simulink model "accTests"  (R2019a)
settings: Solver=VariableStepAuto  StartTime=0.0  StopTime=25  RelTol=1e-3
libraries: simulink x21, autolibshared x5
(part 1 of 2)
settings Model: Creator=Fernando VM  LastModifiedBy=fvall
settings DataIOCC: ReturnWorkspaceOutputs=off
settings DebuggingCC: ArithmeticOperatorsInVariantConditions=warning

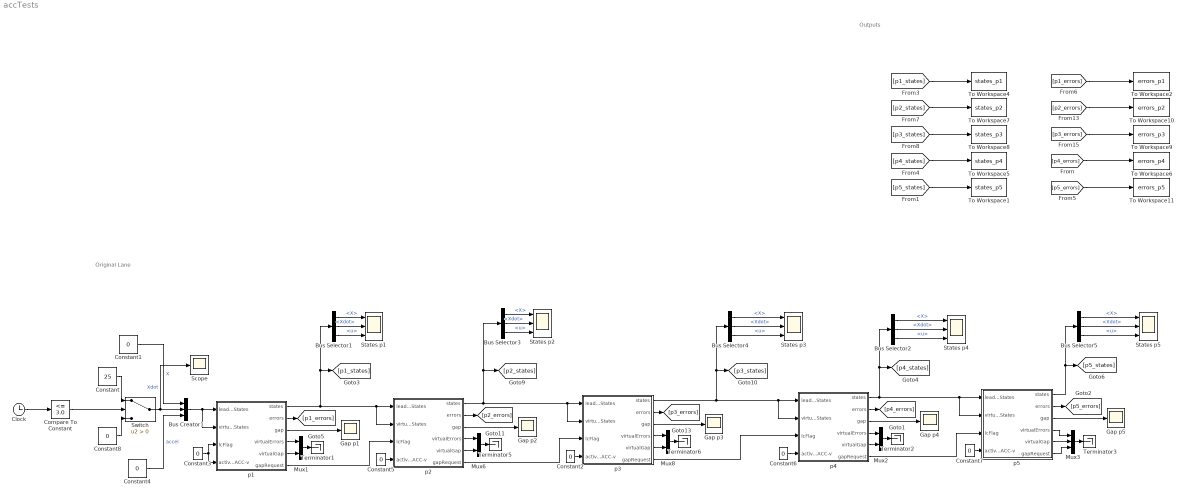
== system accTests ==
  note: Original Lane
  note: Outputs
  Bus Creator1 : BusCreator  Inputs=3
  Bus Selector{1..5} (5 alike) : BusSelector  OutputSignals=X,Xdot,u
  Clock : Clock
  Compare To Constant : simulink/Logic and Bit Operations/Compare To Constant  relop=<=  const=3.0  OutDataTypeStr=boolean
  Constant : Constant  Value=25
  Constant{1..8} (8 alike) : Constant  Value=0
  Gap p{1..5} (5 alike) : Scope
  Mux{1..2,6,8} (4 alike) : Mux  Inputs=2
  Mux3 : Mux  Inputs=3
  Scope : Scope
  States p{1..5} (5 alike) : Scope  NumInputPorts=3
  Switch : Switch  Criteria=u2 > Threshold
  Terminator{1..3,5..6} (5 alike) : Terminator
  To Workspace1 : ToWorkspace  VariableName=states_p5  SampleTime=-1
  To Workspace10 : ToWorkspace  VariableName=errors_p2  SampleTime=-1
  To Workspace11 : ToWorkspace  VariableName=errors_p5  SampleTime=-1
  To Workspace2 : ToWorkspace  VariableName=errors_p1  SampleTime=-1
  To Workspace4 : ToWorkspace  VariableName=states_p1  SampleTime=-1
  To Workspace5 : ToWorkspace  VariableName=states_p4  SampleTime=-1
  To Workspace6 : ToWorkspace  VariableName=errors_p4  SampleTime=-1
  To Workspace7 : ToWorkspace  VariableName=states_p2  SampleTime=-1
  To Workspace8 : ToWorkspace  VariableName=states_p3  SampleTime=-1
  To Workspace9 : ToWorkspace  VariableName=errors_p3  SampleTime=-1
  p1 : Subsystem  mask{m=2000, lf=2.5, lr=2.5, maxAcceleration=4, minAcceleration=-8, maxJerk=40, minJerk=-40, x0=87.76, vx0=25, y0=0, h=0.66, hLc=0.88, d0=0.44, d0Lc=0.44, minHeadwayError=-100, maxHeadwayError=3, velFilterGain=10, Kd=1.3536, Kp=7.04, Ki=6, velKi=0.5, velKp=1.5, vMin=18}
      mask prompts: m "autoblks_shared:autoblkVehBody3DofLat:blkPrm_m"; lf "autoblks_shared:autoblkVehBody3DofLat:blkPrm_a"; lr "autoblks_shared:autoblkVehBody3DofLat:blkPrm_b"; maxAcceleration "Max Acceleration"; minAcceleration "Min Acceleration"; maxJerk "Max Jerk"; minJerk "Min Jerk"; x0 "autoblks_shared:autoblkVehBody3DofLat:blkPrm_X_o"; vx0 "autoblks_shared:autoblkVehBody3DofLat:blkPrm_xdot_o"; y0 "autoblks_shared:autoblkVehBody3DofLat:blkPrm_Y_o"; h "Time Headway"; hLc "Time Headway LC"; d0 "Standstill Gap"; d0Lc "Standstill Gap LC"; minHeadwayError "Min Headway Error"; maxHeadwayError "Max Headway Error"; velFilterGain "Velocity Filter Gain"; vMin "Min Gap Gen Speed"
      mask TypeOptions m: Vehicle Body 3DOF Single Track/m
      mask TypeOptions lf: Vehicle Body 3DOF Single Track/a
      mask TypeOptions lr: Vehicle Body 3DOF Single Track/b
      mask TypeOptions x0: Vehicle Body 3DOF Single Track/X_o
      mask TypeOptions vx0: Vehicle Body 3DOF Single Track/xdot_o
      mask TypeOptions y0: Vehicle Body 3DOF Single Track/Y_o
      mask TypeOptions h: ACC/Headway error/h/Value
      mask TypeOptions hLc: ACC/Headway error/hLc/Value
      mask TypeOptions d0: ACC/Headway error/d0/Value
      mask TypeOptions d0Lc: ACC/Headway error/d0Lc/Value
      mask TypeOptions Kd: ACC/Kd/Gain
      mask TypeOptions Kp: ACC/Kp/Gain
      mask TypeOptions Ki: ACC/Ki/Gain
      mask TypeOptions velKi: ACC/velKi/Gain
      mask TypeOptions velKp: ACC/velKp/Gain
      mask TypeOptions vMin: ACC-v/vMin/Value
      mask DialogControl DescGroupVar Prompt: 3DOF Vehicle with ACC
      mask DialogControl DescTextVar Prompt: Vehicle with ACC. The vehicle model is Simulink's 3DOF single track vehicle body. The controller is a PID with constant headway including headway error saturation and filtered leader velocity.
      mask DialogControl ParameterGroupVar Prompt: Vehicle Parameters
      mask DialogControl m Prompt: Vehicle mass, m [kg]:
      mask DialogControl lf Prompt: Longitudinal distance from center of mass to front axle, a [m]:
      mask DialogControl lr Prompt: Longitudinal distance from center of mass to rear axle, b [m]:
      mask DialogControl x0 Prompt: Initial inertial frame longitudinal position, X_o [m]:
      mask DialogControl vx0 Prompt: Initial longitudinal velocity, xdot_o [m/s]:
      mask DialogControl y0 Prompt: Initial inertial frame lateral displacement, Y_o [m]:
      mask DialogControl Container3 Prompt: Controller Parameters
  p2 : Subsystem  mask{m=2000, lf=2.5, lr=2.5, maxAcceleration=4, minAcceleration=-8, maxJerk=40, minJerk=-40, x0=65.82, vx0=25, y0=0, h=0.66, hLc=0.88, d0=0.44, d0Lc=0.44, minHeadwayError=-100, maxHeadwayError=3, velFilterGain=10, Kd=1.3536, Kp=7.04, Ki=6, velKi=0.5, velKp=1.5, vMin=18}
      mask prompts: m "autoblks_shared:autoblkVehBody3DofLat:blkPrm_m"; lf "autoblks_shared:autoblkVehBody3DofLat:blkPrm_a"; lr "autoblks_shared:autoblkVehBody3DofLat:blkPrm_b"; maxAcceleration "Max Acceleration"; minAcceleration "Min Acceleration"; maxJerk "Max Jerk"; minJerk "Min Jerk"; x0 "autoblks_shared:autoblkVehBody3DofLat:blkPrm_X_o"; vx0 "autoblks_shared:autoblkVehBody3DofLat:blkPrm_xdot_o"; y0 "autoblks_shared:autoblkVehBody3DofLat:blkPrm_Y_o"; h "Time Headway"; hLc "Time Headway LC"; d0 "Standstill Gap"; d0Lc "Standstill Gap LC"; minHeadwayError "Min Headway Error"; maxHeadwayError "Max Headway Error"; velFilterGain "Velocity Filter Gain"; vMin "Min Gap Gen Speed"
      mask TypeOptions m: Vehicle Body 3DOF Single Track/m
      mask TypeOptions lf: Vehicle Body 3DOF Single Track/a
      mask TypeOptions lr: Vehicle Body 3DOF Single Track/b
      mask TypeOptions x0: Vehicle Body 3DOF Single Track/X_o
      mask TypeOptions vx0: Vehicle Body 3DOF Single Track/xdot_o
      mask TypeOptions y0: Vehicle Body 3DOF Single Track/Y_o
      mask TypeOptions h: ACC/Headway error/h/Value
      mask TypeOptions hLc: ACC/Headway error/hLc/Value
      mask TypeOptions d0: ACC/Headway error/d0/Value
      mask TypeOptions d0Lc: ACC/Headway error/d0Lc/Value
      mask TypeOptions Kd: ACC/Kd/Gain
      mask TypeOptions Kp: ACC/Kp/Gain
      mask TypeOptions Ki: ACC/Ki/Gain
      mask TypeOptions velKi: ACC/velKi/Gain
      mask TypeOptions velKp: ACC/velKp/Gain
      mask TypeOptions vMin: ACC-v/vMin/Value
      mask DialogControl DescGroupVar Prompt: 3DOF Vehicle with ACC
      mask DialogControl DescTextVar Prompt: Vehicle with ACC. The vehicle model is Simulink's 3DOF single track vehicle body. The controller is a PID with constant headway including headway error saturation and filtered leader velocity.
      mask DialogControl ParameterGroupVar Prompt: Vehicle Parameters
      mask DialogControl m Prompt: Vehicle mass, m [kg]:
      mask DialogControl lf Prompt: Longitudinal distance from center of mass to front axle, a [m]:
      mask DialogControl lr Prompt: Longitudinal distance from center of mass to rear axle, b [m]:
      mask DialogControl x0 Prompt: Initial inertial frame longitudinal position, X_o [m]:
      mask DialogControl vx0 Prompt: Initial longitudinal velocity, xdot_o [m/s]:
      mask DialogControl y0 Prompt: Initial inertial frame lateral displacement, Y_o [m]:
      mask DialogControl Container3 Prompt: Controller Parameters
  p3 : Subsystem  mask{m=2000, lf=2.5, lr=2.5, maxAcceleration=4, minAcceleration=-8, maxJerk=40, minJerk=-40, x0=43.88, vx0=25, y0=0, h=0.66, hLc=0.88, d0=0.44, d0Lc=0.44, minHeadwayError=-100, maxHeadwayError=3, velFilterGain=10, Kd=1.3536, Kp=7.04, Ki=6, velKi=0.5, velKp=1.5, vMin=18}
      mask prompts: m "autoblks_shared:autoblkVehBody3DofLat:blkPrm_m"; lf "autoblks_shared:autoblkVehBody3DofLat:blkPrm_a"; lr "autoblks_shared:autoblkVehBody3DofLat:blkPrm_b"; maxAcceleration "Max Acceleration"; minAcceleration "Min Acceleration"; maxJerk "Max Jerk"; minJerk "Min Jerk"; x0 "autoblks_shared:autoblkVehBody3DofLat:blkPrm_X_o"; vx0 "autoblks_shared:autoblkVehBody3DofLat:blkPrm_xdot_o"; y0 "autoblks_shared:autoblkVehBody3DofLat:blkPrm_Y_o"; h "Time Headway"; hLc "Time Headway LC"; d0 "Standstill Gap"; d0Lc "Standstill Gap LC"; minHeadwayError "Min Headway Error"; maxHeadwayError "Max Headway Error"; velFilterGain "Velocity Filter Gain"; vMin "Min Gap Gen Speed"
      mask TypeOptions m: Vehicle Body 3DOF Single Track/m
      mask TypeOptions lf: Vehicle Body 3DOF Single Track/a
      mask TypeOptions lr: Vehicle Body 3DOF Single Track/b
      mask TypeOptions x0: Vehicle Body 3DOF Single Track/X_o
      mask TypeOptions vx0: Vehicle Body 3DOF Single Track/xdot_o
      mask TypeOptions y0: Vehicle Body 3DOF Single Track/Y_o
      mask TypeOptions h: ACC/Headway error/h/Value
      mask TypeOptions hLc: ACC/Headway error/hLc/Value
      mask TypeOptions d0: ACC/Headway error/d0/Value
      mask TypeOptions d0Lc: ACC/Headway error/d0Lc/Value
      mask TypeOptions Kd: ACC/Kd/Gain
      mask TypeOptions Kp: ACC/Kp/Gain
      mask TypeOptions Ki: ACC/Ki/Gain
      mask TypeOptions velKi: ACC/velKi/Gain
      mask TypeOptions velKp: ACC/velKp/Gain
      mask TypeOptions vMin: ACC-v/vMin/Value
      mask DialogControl DescGroupVar Prompt: 3DOF Vehicle with ACC
      mask DialogControl DescTextVar Prompt: Vehicle with ACC. The vehicle model is Simulink's 3DOF single track vehicle body. The controller is a PID with constant headway including headway error saturation and filtered leader velocity.
      mask DialogControl ParameterGroupVar Prompt: Vehicle Parameters
      mask DialogControl m Prompt: Vehicle mass, m [kg]:
      mask DialogControl lf Prompt: Longitudinal distance from center of mass to front axle, a [m]:
      mask DialogControl lr Prompt: Longitudinal distance from center of mass to rear axle, b [m]:
      mask DialogControl x0 Prompt: Initial inertial frame longitudinal position, X_o [m]:
      mask DialogControl vx0 Prompt: Initial longitudinal velocity, xdot_o [m/s]:
      mask DialogControl y0 Prompt: Initial inertial frame lateral displacement, Y_o [m]:
      mask DialogControl Container3 Prompt: Controller Parameters
  p4 : Subsystem  mask{m=2000, lf=2.5, lr=2.5, maxAcceleration=4, minAcceleration=-8, maxJerk=40, minJerk=-40, x0=21.94, vx0=25, y0=0, h=0.66, hLc=0.88, d0=0.44, d0Lc=0.44, minHeadwayError=-100, maxHeadwayError=3, velFilterGain=10, Kd=1.3536, Kp=7.04, Ki=6, velKi=0.5, velKp=1.5, vMin=18}
      mask prompts: m "autoblks_shared:autoblkVehBody3DofLat:blkPrm_m"; lf "autoblks_shared:autoblkVehBody3DofLat:blkPrm_a"; lr "autoblks_shared:autoblkVehBody3DofLat:blkPrm_b"; maxAcceleration "Max Acceleration"; minAcceleration "Min Acceleration"; maxJerk "Max Jerk"; minJerk "Min Jerk"; x0 "autoblks_shared:autoblkVehBody3DofLat:blkPrm_X_o"; vx0 "autoblks_shared:autoblkVehBody3DofLat:blkPrm_xdot_o"; y0 "autoblks_shared:autoblkVehBody3DofLat:blkPrm_Y_o"; h "Time Headway"; hLc "Time Headway LC"; d0 "Standstill Gap"; d0Lc "Standstill Gap LC"; minHeadwayError "Min Headway Error"; maxHeadwayError "Max Headway Error"; velFilterGain "Velocity Filter Gain"; vMin "Min Gap Gen Speed"
      mask TypeOptions m: Vehicle Body 3DOF Single Track/m
      mask TypeOptions lf: Vehicle Body 3DOF Single Track/a
      mask TypeOptions lr: Vehicle Body 3DOF Single Track/b
      mask TypeOptions x0: Vehicle Body 3DOF Single Track/X_o
      mask TypeOptions vx0: Vehicle Body 3DOF Single Track/xdot_o
      mask TypeOptions y0: Vehicle Body 3DOF Single Track/Y_o
      mask TypeOptions h: ACC/Headway error/h/Value
      mask TypeOptions hLc: ACC/Headway error/hLc/Value
      mask TypeOptions d0: ACC/Headway error/d0/Value
      mask TypeOptions d0Lc: ACC/Headway error/d0Lc/Value
      mask TypeOptions Kd: ACC/Kd/Gain
      mask TypeOptions Kp: ACC/Kp/Gain
      mask TypeOptions Ki: ACC/Ki/Gain
      mask TypeOptions velKi: ACC/velKi/Gain
      mask TypeOptions velKp: ACC/velKp/Gain
      mask TypeOptions vMin: ACC-v/vMin/Value
      mask DialogControl DescGroupVar Prompt: 3DOF Vehicle with ACC
      mask DialogControl DescTextVar Prompt: Vehicle with ACC. The vehicle model is Simulink's 3DOF single track vehicle body. The controller is a PID with constant headway including headway error saturation and filtered leader velocity.
      mask DialogControl ParameterGroupVar Prompt: Vehicle Parameters
      mask DialogControl m Prompt: Vehicle mass, m [kg]:
      mask DialogControl lf Prompt: Longitudinal distance from center of mass to front axle, a [m]:
      mask DialogControl lr Prompt: Longitudinal distance from center of mass to rear axle, b [m]:
      mask DialogControl x0 Prompt: Initial inertial frame longitudinal position, X_o [m]:
      mask DialogControl vx0 Prompt: Initial longitudinal velocity, xdot_o [m/s]:
      mask DialogControl y0 Prompt: Initial inertial frame lateral displacement, Y_o [m]:
      mask DialogControl Container3 Prompt: Controller Parameters
  p5 : Subsystem  mask{m=2000, lf=2.5, lr=2.5, maxAcceleration=4, minAcceleration=-8, maxJerk=40, minJerk=-40, x0=0, vx0=25, y0=0, h=0.66, hLc=0.88, d0=0.44, d0Lc=0.44, minHeadwayError=-100, maxHeadwayError=3, velFilterGain=10, Kd=1.3536, Kp=7.04, Ki=6, velKi=0.5, velKp=1.5, vMin=18}
      mask prompts: m "autoblks_shared:autoblkVehBody3DofLat:blkPrm_m"; lf "autoblks_shared:autoblkVehBody3DofLat:blkPrm_a"; lr "autoblks_shared:autoblkVehBody3DofLat:blkPrm_b"; maxAcceleration "Max Acceleration"; minAcceleration "Min Acceleration"; maxJerk "Max Jerk"; minJerk "Min Jerk"; x0 "autoblks_shared:autoblkVehBody3DofLat:blkPrm_X_o"; vx0 "autoblks_shared:autoblkVehBody3DofLat:blkPrm_xdot_o"; y0 "autoblks_shared:autoblkVehBody3DofLat:blkPrm_Y_o"; h "Time Headway"; hLc "Time Headway LC"; d0 "Standstill Gap"; d0Lc "Standstill Gap LC"; minHeadwayError "Min Headway Error"; maxHeadwayError "Max Headway Error"; velFilterGain "Velocity Filter Gain"; vMin "Min Gap Gen Speed"
      mask TypeOptions m: Vehicle Body 3DOF Single Track/m
      mask TypeOptions lf: Vehicle Body 3DOF Single Track/a
      mask TypeOptions lr: Vehicle Body 3DOF Single Track/b
      mask TypeOptions x0: Vehicle Body 3DOF Single Track/X_o
      mask TypeOptions vx0: Vehicle Body 3DOF Single Track/xdot_o
      mask TypeOptions y0: Vehicle Body 3DOF Single Track/Y_o
      mask TypeOptions h: ACC/Headway error/h/Value
      mask TypeOptions hLc: ACC/Headway error/hLc/Value
      mask TypeOptions d0: ACC/Headway error/d0/Value
      mask TypeOptions d0Lc: ACC/Headway error/d0Lc/Value
      mask TypeOptions Kd: ACC/Kd/Gain
      mask TypeOptions Kp: ACC/Kp/Gain
      mask TypeOptions Ki: ACC/Ki/Gain
      mask TypeOptions velKi: ACC/velKi/Gain
      mask TypeOptions velKp: ACC/velKp/Gain
      mask TypeOptions vMin: ACC-v/vMin/Value
      mask DialogControl DescGroupVar Prompt: 3DOF Vehicle with ACC
      mask DialogControl DescTextVar Prompt: Vehicle with ACC. The vehicle model is Simulink's 3DOF single track vehicle body. The controller is a PID with constant headway including headway error saturation and filtered leader velocity.
      mask DialogControl ParameterGroupVar Prompt: Vehicle Parameters
      mask DialogControl m Prompt: Vehicle mass, m [kg]:
      mask DialogControl lf Prompt: Longitudinal distance from center of mass to front axle, a [m]:
      mask DialogControl lr Prompt: Longitudinal distance from center of mass to rear axle, b [m]:
      mask DialogControl x0 Prompt: Initial inertial frame longitudinal position, X_o [m]:
      mask DialogControl vx0 Prompt: Initial longitudinal velocity, xdot_o [m/s]:
      mask DialogControl y0 Prompt: Initial inertial frame lateral displacement, Y_o [m]:
      mask DialogControl Container3 Prompt: Controller Parameters
  wires:
  p2/6(gapRequest) -> p3/3(lcFlag)
  Bus Selector4/2 -> States p3/2  "<Xdot>"
  Bus Selector1/2 -> States p1/2  "<Xdot>"
  p2/4(virtualErrors) -> Mux6/1
  Mux8/1 -> Terminator6/1
  p3/3(gap) -> Gap p3/1
  Bus Selector1/3 -> States p1/3  "<u>"
  p2/3(gap) -> Gap p2/1
  Constant5/1 -> p2/4(activate ACC-v)
  p3/4(virtualErrors) -> Mux8/1
  p2/5(virtualGap) -> Mux6/2
  p3/5(virtualGap) -> Mux8/2
  Constant2/1 -> p3/4(activate ACC-v)
  p4/3(gap) -> Gap p4/1
  Bus Selector1/1 -> States p1/1  "<X>"
  Mux6/1 -> Terminator5/1
  p3/1(states) -> p4/1(leaderStates), p4/2(virtualLeaderStates), Bus Selector4/1, [p3_states]
  p1/2(errors) -> [p1_errors]
  Constant4/1 -> Bus Creator1/3  "accel"
  p1/1(states) -> Bus Selector1/1, [p1_states], p2/2(virtualLeaderStates), p2/1(leaderStates)
  p2/1(states) -> p3/1(leaderStates), p3/2(virtualLeaderStates), [p2_states], Bus Selector3/1
  Bus Creator1/1 -> p1/2(virtualLeaderStates), p1/1(leaderStates)
  Constant1/1 -> Bus Creator1/1  "X"
  Switch/1 -> Scope/1, Bus Creator1/2  "Xdot"
  p1/6(gapRequest) -> p2/3(lcFlag)
  Bus Selector3/2 -> States p2/2  "<Xdot>"
  p3/2(errors) -> [p3_errors]
  p2/2(errors) -> [p2_errors]
  Bus Selector4/1 -> States p3/1  "<X>"
  Bus Selector3/3 -> States p2/3  "<u>"
  Bus Selector3/1 -> States p2/1  "<X>"
  Bus Selector4/3 -> States p3/3  "<u>"
  [p4_states] -> To Workspace5/1
  [p2_states] -> To Workspace7/1
  [p1_errors] -> To Workspace2/1
  [p1_states] -> To Workspace4/1
  [p4_errors] -> To Workspace6/1
  [p3_states] -> To Workspace8/1
  [p2_errors] -> To Workspace10/1
  [p3_errors] -> To Workspace9/1
  Constant3/1 -> p1/4(activate ACC-v), p1/3(lcFlag)
  Constant6/1 -> p4/4(activate ACC-v)
  p3/6(gapRequest) -> p4/3(lcFlag)
  p1/3(gap) -> Gap p1/1
  Mux1/1 -> Terminator1/1
  p1/5(virtualGap) -> Mux1/2
  p1/4(virtualErrors) -> Mux1/1
  p4/2(errors) -> [p4_errors]
  Bus Selector2/3 -> States p4/3  "<u>"
  Bus Selector2/1 -> States p4/1  "<X>"
  Bus Selector2/2 -> States p4/2  "<Xdot>"
  p4/5(virtualGap) -> Mux2/2
  p4/4(virtualErrors) -> Mux2/1
  Mux2/1 -> Terminator2/1
  p5/5(virtualGap) -> Mux3/2
  p5/4(virtualErrors) -> Mux3/1
  p4/6(gapRequest) -> p5/3(lcFlag)
  Constant7/1 -> p5/4(activate ACC-v)
  p5/2(errors) -> [p5_errors]
  Mux3/1 -> Terminator3/1
  Bus Selector5/1 -> States p5/1  "<X>"
  Bus Selector5/2 -> States p5/2  "<Xdot>"
  p5/1(states) -> Bus Selector5/1, [p5_states]
  Bus Selector5/3 -> States p5/3  "<u>"
  p5/3(gap) -> Gap p5/1
  p4/1(states) -> p5/2(virtualLeaderStates), p5/1(leaderStates), Bus Selector2/1, [p4_states]
  [p5_states] -> To Workspace1/1
  [p5_errors] -> To Workspace11/1
  Constant/1 -> Switch/1
  Constant8/1 -> Switch/3
  Clock/1 -> Compare To Constant/1
  Compare To Constant/1 -> Switch/2
  p5/6(gapRequest) -> Mux3/3

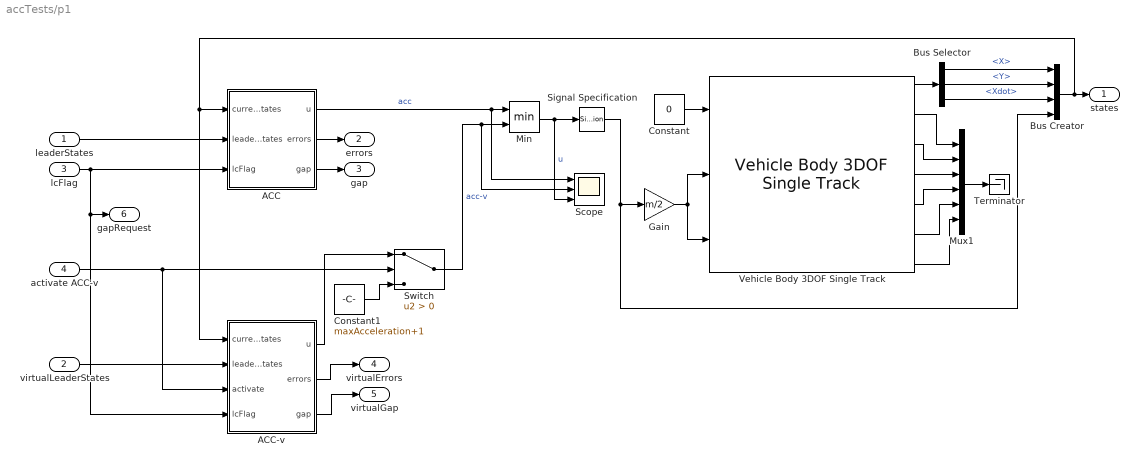
== system accTests/p1 ==
  leaderStates : Inport
  virtualLeaderStates : Inport  Port=2
  lcFlag : Inport  Port=3
  activate ACC-v : Inport  Port=4
  ACC : Subsystem
  ACC-v : Subsystem
  Bus Creator : BusCreator  Inputs=4
  Bus Selector : BusSelector  OutputSignals=InertFrm.RearAxl.Disp.X,InertFrm.RearAxl.Disp.Y,InertFrm.RearAxl.Vel.Xdot
  Constant : Constant  Value=0
  Constant1 : Constant  Value=maxAcceleration+1
  Gain : Gain  Gain=m/2
  Min : MinMax  Inputs=2
  Mux1 : Mux  Inputs=6
  Scope : Scope  NumInputPorts=3
  Signal Specification : SignalSpecification  Dimensions=1
  Switch : Switch  Criteria=u2 > Threshold
  Terminator : Terminator
  Vehicle Body 3DOF Single Track : autolibshared/Vehicle Body 3DOF Single Track  trackMode=Single (bicycle)  inputMode=External longitudinal forces  frontSteerMode=on  rearSteerMode=off  windMode=off  muMode=off  extFMode=off  extMMode=off  extXo=off  extpsio=off  extxdoto=off  extro=off  extYo=off  extTamb=off  extydoto=off  aMode=2  NF=2  NR=2  m=m  a=lf  b=lr  h=0.35  X_o=x0  xdot_o=vx0  CalphaMode=off  sigmaMode=on  d=0  w=[1.4,1.4]  Cy_f=12e3  Cy_r=11e3  sigma_f=.1  sigma_r=.1  alpha_f_brk=[-.1 .1]  Cy_f_data=[-9e3 9e3]  alpha_r_brk=[-.1 .1]  Cy_r_data=[-9e3 9e3]  Y_o=y0  ydot_o=0  Izz=4000  psi_o=0  r_o=0  Af=2  Cd=.3  Cl=.1  Cpm=.1  beta_w=[0:0.01:0.3]  Cs=[0:0.03:0.9]  Cym=[0:0.01:0.3]  Pabs=101325  Tair=273  g=9.81  mu=1  xdot_tol=.01  Fznom=5000  Fxtire_sat=7e4  Fytire_sat=7e4  longOff=0  latOff=0  vertOff=0  wrapAng=off
      settings: SourceProductName=Powertrain Blockset  SourceProductBaseCode=PW
  states : Outport
  errors : Outport  Port=2
  gap : Outport  Port=3
  virtualErrors : Outport  Port=4
  virtualGap : Outport  Port=5
  gapRequest : Outport  Port=6
  wires:
  Bus Selector/3 -> Bus Creator/3  "<Xdot>"
  Bus Selector/1 -> Bus Creator/1  "<X>"
  Min/1 -> Scope/3, Signal Specification/1  "u"
  ACC/1(u) -> Scope/1, Min/1  "acc"
  Gain/1 -> Vehicle Body 3DOF Single Track/3, Vehicle Body 3DOF Single Track/2
  Constant/1 -> Vehicle Body 3DOF Single Track/1
  Vehicle Body 3DOF Single Track/1 -> Bus Selector/1
  Vehicle Body 3DOF Single Track/4 -> Mux1/3
  Vehicle Body 3DOF Single Track/3 -> Mux1/2
  Vehicle Body 3DOF Single Track/2 -> Mux1/1
  Vehicle Body 3DOF Single Track/5 -> Mux1/4
  Vehicle Body 3DOF Single Track/6 -> Mux1/5
  Vehicle Body 3DOF Single Track/7 -> Mux1/6
  Mux1/1 -> Terminator/1
  ACC/3(gap) -> gap/1
  Bus Creator/1 -> ACC/1(currentStates), ACC-v/1(currentStates), states/1
  leaderStates/1 -> ACC/2(leaderStates)
  virtualLeaderStates/1 -> ACC-v/2(leaderStates)
  ACC/2(errors) -> errors/1
  lcFlag/1 -> ACC-v/4(lcFlag), gapRequest/1, ACC/3(lcFlag)
  Switch/1 -> Scope/2, Min/2  "acc-v"
  ACC-v/1(u) -> Switch/1
  ACC-v/2(errors) -> virtualErrors/1
  ACC-v/3(gap) -> virtualGap/1
  Bus Selector/2 -> Bus Creator/2  "<Y>"
  Signal Specification/1 -> Bus Creator/4, Gain/1
  activate ACC-v/1 -> ACC-v/3(activate), Switch/2
  Constant1/1 -> Switch/3

== system accTests/p2 ==
  leaderStates : Inport
  virtualLeaderStates : Inport  Port=2
  lcFlag : Inport  Port=3
  activate ACC-v : Inport  Port=4
  ACC : Subsystem
  ACC-v : Subsystem
  Bus Creator : BusCreator  Inputs=4
  Bus Selector : BusSelector  OutputSignals=InertFrm.RearAxl.Disp.X,InertFrm.RearAxl.Disp.Y,InertFrm.RearAxl.Vel.Xdot
  Constant : Constant  Value=0
  Constant1 : Constant  Value=maxAcceleration+1
  Gain : Gain  Gain=m/2
  Min : MinMax  Inputs=2
  Mux1 : Mux  Inputs=6
  Scope : Scope  NumInputPorts=3
  Signal Specification : SignalSpecification  Dimensions=1
  Switch : Switch  Criteria=u2 > Threshold
  Terminator : Terminator
  Vehicle Body 3DOF Single Track : autolibshared/Vehicle Body 3DOF Single Track  trackMode=Single (bicycle)  inputMode=External longitudinal forces  frontSteerMode=on  rearSteerMode=off  windMode=off  muMode=off  extFMode=off  extMMode=off  extXo=off  extpsio=off  extxdoto=off  extro=off  extYo=off  extTamb=off  extydoto=off  aMode=2  NF=2  NR=2  m=m  a=lf  b=lr  h=0.35  X_o=x0  xdot_o=vx0  CalphaMode=off  sigmaMode=on  d=0  w=[1.4,1.4]  Cy_f=12e3  Cy_r=11e3  sigma_f=.1  sigma_r=.1  alpha_f_brk=[-.1 .1]  Cy_f_data=[-9e3 9e3]  alpha_r_brk=[-.1 .1]  Cy_r_data=[-9e3 9e3]  Y_o=y0  ydot_o=0  Izz=4000  psi_o=0  r_o=0  Af=2  Cd=.3  Cl=.1  Cpm=.1  beta_w=[0:0.01:0.3]  Cs=[0:0.03:0.9]  Cym=[0:0.01:0.3]  Pabs=101325  Tair=273  g=9.81  mu=1  xdot_tol=.01  Fznom=5000  Fxtire_sat=7e4  Fytire_sat=7e4  longOff=0  latOff=0  vertOff=0  wrapAng=off
      settings: SourceProductName=Powertrain Blockset  SourceProductBaseCode=PW
  states : Outport
  errors : Outport  Port=2
  gap : Outport  Port=3
  virtualErrors : Outport  Port=4
  virtualGap : Outport  Port=5
  gapRequest : Outport  Port=6
  wires:
  Bus Selector/3 -> Bus Creator/3  "<Xdot>"
  Bus Selector/1 -> Bus Creator/1  "<X>"
  Min/1 -> Scope/3, Signal Specification/1  "u"
  ACC/1(u) -> Scope/1, Min/1  "acc"
  Gain/1 -> Vehicle Body 3DOF Single Track/3, Vehicle Body 3DOF Single Track/2
  Constant/1 -> Vehicle Body 3DOF Single Track/1
  Vehicle Body 3DOF Single Track/1 -> Bus Selector/1
  Vehicle Body 3DOF Single Track/4 -> Mux1/3
  Vehicle Body 3DOF Single Track/3 -> Mux1/2
  Vehicle Body 3DOF Single Track/2 -> Mux1/1
  Vehicle Body 3DOF Single Track/5 -> Mux1/4
  Vehicle Body 3DOF Single Track/6 -> Mux1/5
  Vehicle Body 3DOF Single Track/7 -> Mux1/6
  Mux1/1 -> Terminator/1
  ACC/3(gap) -> gap/1
  Bus Creator/1 -> ACC/1(currentStates), ACC-v/1(currentStates), states/1
  leaderStates/1 -> ACC/2(leaderStates)
  virtualLeaderStates/1 -> ACC-v/2(leaderStates)
  ACC/2(errors) -> errors/1
  lcFlag/1 -> ACC-v/4(lcFlag), gapRequest/1, ACC/3(lcFlag)
  Switch/1 -> Scope/2, Min/2  "acc-v"
  ACC-v/1(u) -> Switch/1
  ACC-v/2(errors) -> virtualErrors/1
  ACC-v/3(gap) -> virtualGap/1
  Bus Selector/2 -> Bus Creator/2  "<Y>"
  Signal Specification/1 -> Bus Creator/4, Gain/1
  activate ACC-v/1 -> ACC-v/3(activate), Switch/2
  Constant1/1 -> Switch/3

== system accTests/p3 ==
  leaderStates : Inport
  virtualLeaderStates : Inport  Port=2
  lcFlag : Inport  Port=3
  activate ACC-v : Inport  Port=4
  ACC : Subsystem
  ACC-v : Subsystem
  Bus Creator : BusCreator  Inputs=4
  Bus Selector : BusSelector  OutputSignals=InertFrm.RearAxl.Disp.X,InertFrm.RearAxl.Disp.Y,InertFrm.RearAxl.Vel.Xdot
  Constant : Constant  Value=0
  Constant1 : Constant  Value=maxAcceleration+1
  Gain : Gain  Gain=m/2
  Min : MinMax  Inputs=2
  Mux1 : Mux  Inputs=6
  Scope : Scope  NumInputPorts=3
  Signal Specification : SignalSpecification  Dimensions=1
  Switch : Switch  Criteria=u2 > Threshold
  Terminator : Terminator
  Vehicle Body 3DOF Single Track : autolibshared/Vehicle Body 3DOF Single Track  trackMode=Single (bicycle)  inputMode=External longitudinal forces  frontSteerMode=on  rearSteerMode=off  windMode=off  muMode=off  extFMode=off  extMMode=off  extXo=off  extpsio=off  extxdoto=off  extro=off  extYo=off  extTamb=off  extydoto=off  aMode=2  NF=2  NR=2  m=m  a=lf  b=lr  h=0.35  X_o=x0  xdot_o=vx0  CalphaMode=off  sigmaMode=on  d=0  w=[1.4,1.4]  Cy_f=12e3  Cy_r=11e3  sigma_f=.1  sigma_r=.1  alpha_f_brk=[-.1 .1]  Cy_f_data=[-9e3 9e3]  alpha_r_brk=[-.1 .1]  Cy_r_data=[-9e3 9e3]  Y_o=y0  ydot_o=0  Izz=4000  psi_o=0  r_o=0  Af=2  Cd=.3  Cl=.1  Cpm=.1  beta_w=[0:0.01:0.3]  Cs=[0:0.03:0.9]  Cym=[0:0.01:0.3]  Pabs=101325  Tair=273  g=9.81  mu=1  xdot_tol=.01  Fznom=5000  Fxtire_sat=7e4  Fytire_sat=7e4  longOff=0  latOff=0  vertOff=0  wrapAng=off
      settings: SourceProductName=Powertrain Blockset  SourceProductBaseCode=PW
  states : Outport
  errors : Outport  Port=2
  gap : Outport  Port=3
  virtualErrors : Outport  Port=4
  virtualGap : Outport  Port=5
  gapRequest : Outport  Port=6
  wires:
  Bus Selector/3 -> Bus Creator/3  "<Xdot>"
  Bus Selector/1 -> Bus Creator/1  "<X>"
  Min/1 -> Scope/3, Signal Specification/1  "u"
  ACC/1(u) -> Scope/1, Min/1  "acc"
  Gain/1 -> Vehicle Body 3DOF Single Track/3, Vehicle Body 3DOF Single Track/2
  Constant/1 -> Vehicle Body 3DOF Single Track/1
  Vehicle Body 3DOF Single Track/1 -> Bus Selector/1
  Vehicle Body 3DOF Single Track/4 -> Mux1/3
  Vehicle Body 3DOF Single Track/3 -> Mux1/2
  Vehicle Body 3DOF Single Track/2 -> Mux1/1
  Vehicle Body 3DOF Single Track/5 -> Mux1/4
  Vehicle Body 3DOF Single Track/6 -> Mux1/5
  Vehicle Body 3DOF Single Track/7 -> Mux1/6
  Mux1/1 -> Terminator/1
  ACC/3(gap) -> gap/1
  Bus Creator/1 -> ACC/1(currentStates), ACC-v/1(currentStates), states/1
  leaderStates/1 -> ACC/2(leaderStates)
  virtualLeaderStates/1 -> ACC-v/2(leaderStates)
  ACC/2(errors) -> errors/1
  lcFlag/1 -> ACC-v/4(lcFlag), gapRequest/1, ACC/3(lcFlag)
  Switch/1 -> Scope/2, Min/2  "acc-v"
  ACC-v/1(u) -> Switch/1
  ACC-v/2(errors) -> virtualErrors/1
  ACC-v/3(gap) -> virtualGap/1
  Bus Selector/2 -> Bus Creator/2  "<Y>"
  Signal Specification/1 -> Bus Creator/4, Gain/1
  activate ACC-v/1 -> ACC-v/3(activate), Switch/2
  Constant1/1 -> Switch/3

== system accTests/p4 ==
  leaderStates : Inport
  virtualLeaderStates : Inport  Port=2
  lcFlag : Inport  Port=3
  activate ACC-v : Inport  Port=4
  ACC : Subsystem
  ACC-v : Subsystem
  Bus Creator : BusCreator  Inputs=4
  Bus Selector : BusSelector  OutputSignals=InertFrm.RearAxl.Disp.X,InertFrm.RearAxl.Disp.Y,InertFrm.RearAxl.Vel.Xdot
  Constant : Constant  Value=0
  Constant1 : Constant  Value=maxAcceleration+1
  Gain : Gain  Gain=m/2
  Min : MinMax  Inputs=2
  Mux1 : Mux  Inputs=6
  Scope : Scope  NumInputPorts=3
  Signal Specification : SignalSpecification  Dimensions=1
  Switch : Switch  Criteria=u2 > Threshold
  Terminator : Terminator
  Vehicle Body 3DOF Single Track : autolibshared/Vehicle Body 3DOF Single Track  trackMode=Single (bicycle)  inputMode=External longitudinal forces  frontSteerMode=on  rearSteerMode=off  windMode=off  muMode=off  extFMode=off  extMMode=off  extXo=off  extpsio=off  extxdoto=off  extro=off  extYo=off  extTamb=off  extydoto=off  aMode=2  NF=2  NR=2  m=m  a=lf  b=lr  h=0.35  X_o=x0  xdot_o=vx0  CalphaMode=off  sigmaMode=on  d=0  w=[1.4,1.4]  Cy_f=12e3  Cy_r=11e3  sigma_f=.1  sigma_r=.1  alpha_f_brk=[-.1 .1]  Cy_f_data=[-9e3 9e3]  alpha_r_brk=[-.1 .1]  Cy_r_data=[-9e3 9e3]  Y_o=y0  ydot_o=0  Izz=4000  psi_o=0  r_o=0  Af=2  Cd=.3  Cl=.1  Cpm=.1  beta_w=[0:0.01:0.3]  Cs=[0:0.03:0.9]  Cym=[0:0.01:0.3]  Pabs=101325  Tair=273  g=9.81  mu=1  xdot_tol=.01  Fznom=5000  Fxtire_sat=7e4  Fytire_sat=7e4  longOff=0  latOff=0  vertOff=0  wrapAng=off
      settings: SourceProductName=Powertrain Blockset  SourceProductBaseCode=PW
  states : Outport
  errors : Outport  Port=2
  gap : Outport  Port=3
  virtualErrors : Outport  Port=4
  virtualGap : Outport  Port=5
  gapRequest : Outport  Port=6
  wires:
  Bus Selector/3 -> Bus Creator/3  "<Xdot>"
  Bus Selector/1 -> Bus Creator/1  "<X>"
  Min/1 -> Scope/3, Signal Specification/1  "u"
  ACC/1(u) -> Scope/1, Min/1  "acc"
  Gain/1 -> Vehicle Body 3DOF Single Track/3, Vehicle Body 3DOF Single Track/2
  Constant/1 -> Vehicle Body 3DOF Single Track/1
  Vehicle Body 3DOF Single Track/1 -> Bus Selector/1
  Vehicle Body 3DOF Single Track/4 -> Mux1/3
  Vehicle Body 3DOF Single Track/3 -> Mux1/2
  Vehicle Body 3DOF Single Track/2 -> Mux1/1
  Vehicle Body 3DOF Single Track/5 -> Mux1/4
  Vehicle Body 3DOF Single Track/6 -> Mux1/5
  Vehicle Body 3DOF Single Track/7 -> Mux1/6
  Mux1/1 -> Terminator/1
  ACC/3(gap) -> gap/1
  Bus Creator/1 -> ACC/1(currentStates), ACC-v/1(currentStates), states/1
  leaderStates/1 -> ACC/2(leaderStates)
  virtualLeaderStates/1 -> ACC-v/2(leaderStates)
  ACC/2(errors) -> errors/1
  lcFlag/1 -> ACC-v/4(lcFlag), gapRequest/1, ACC/3(lcFlag)
  Switch/1 -> Scope/2, Min/2  "acc-v"
  ACC-v/1(u) -> Switch/1
  ACC-v/2(errors) -> virtualErrors/1
  ACC-v/3(gap) -> virtualGap/1
  Bus Selector/2 -> Bus Creator/2  "<Y>"
  Signal Specification/1 -> Bus Creator/4, Gain/1
  activate ACC-v/1 -> ACC-v/3(activate), Switch/2
  Constant1/1 -> Switch/3

== system accTests/p5 ==
  leaderStates : Inport
  virtualLeaderStates : Inport  Port=2
  lcFlag : Inport  Port=3
  activate ACC-v : Inport  Port=4
  ACC : Subsystem
  ACC-v : Subsystem
  Bus Creator : BusCreator  Inputs=4
  Bus Selector : BusSelector  OutputSignals=InertFrm.RearAxl.Disp.X,InertFrm.RearAxl.Disp.Y,InertFrm.RearAxl.Vel.Xdot
  Constant : Constant  Value=0
  Constant1 : Constant  Value=maxAcceleration+1
  Gain : Gain  Gain=m/2
  Min : MinMax  Inputs=2
  Mux1 : Mux  Inputs=6
  Scope : Scope  NumInputPorts=3
  Signal Specification : SignalSpecification  Dimensions=1
  Switch : Switch  Criteria=u2 > Threshold
  Terminator : Terminator
  Vehicle Body 3DOF Single Track : autolibshared/Vehicle Body 3DOF Single Track  trackMode=Single (bicycle)  inputMode=External longitudinal forces  frontSteerMode=on  rearSteerMode=off  windMode=off  muMode=off  extFMode=off  extMMode=off  extXo=off  extpsio=off  extxdoto=off  extro=off  extYo=off  extTamb=off  extydoto=off  aMode=2  NF=2  NR=2  m=m  a=lf  b=lr  h=0.35  X_o=x0  xdot_o=vx0  CalphaMode=off  sigmaMode=on  d=0  w=[1.4,1.4]  Cy_f=12e3  Cy_r=11e3  sigma_f=.1  sigma_r=.1  alpha_f_brk=[-.1 .1]  Cy_f_data=[-9e3 9e3]  alpha_r_brk=[-.1 .1]  Cy_r_data=[-9e3 9e3]  Y_o=y0  ydot_o=0  Izz=4000  psi_o=0  r_o=0  Af=2  Cd=.3  Cl=.1  Cpm=.1  beta_w=[0:0.01:0.3]  Cs=[0:0.03:0.9]  Cym=[0:0.01:0.3]  Pabs=101325  Tair=273  g=9.81  mu=1  xdot_tol=.01  Fznom=5000  Fxtire_sat=7e4  Fytire_sat=7e4  longOff=0  latOff=0  vertOff=0  wrapAng=off
      settings: SourceProductName=Powertrain Blockset  SourceProductBaseCode=PW
  states : Outport
  errors : Outport  Port=2
  gap : Outport  Port=3
  virtualErrors : Outport  Port=4
  virtualGap : Outport  Port=5
  gapRequest : Outport  Port=6
  wires:
  Bus Selector/3 -> Bus Creator/3  "<Xdot>"
  Bus Selector/1 -> Bus Creator/1  "<X>"
  Min/1 -> Scope/3, Signal Specification/1  "u"
  ACC/1(u) -> Scope/1, Min/1  "acc"
  Gain/1 -> Vehicle Body 3DOF Single Track/3, Vehicle Body 3DOF Single Track/2
  Constant/1 -> Vehicle Body 3DOF Single Track/1
  Vehicle Body 3DOF Single Track/1 -> Bus Selector/1
  Vehicle Body 3DOF Single Track/4 -> Mux1/3
  Vehicle Body 3DOF Single Track/3 -> Mux1/2
  Vehicle Body 3DOF Single Track/2 -> Mux1/1
  Vehicle Body 3DOF Single Track/5 -> Mux1/4
  Vehicle Body 3DOF Single Track/6 -> Mux1/5
  Vehicle Body 3DOF Single Track/7 -> Mux1/6
  Mux1/1 -> Terminator/1
  ACC/3(gap) -> gap/1
  Bus Creator/1 -> ACC/1(currentStates), ACC-v/1(currentStates), states/1
  leaderStates/1 -> ACC/2(leaderStates)
  virtualLeaderStates/1 -> ACC-v/2(leaderStates)
  ACC/2(errors) -> errors/1
  lcFlag/1 -> ACC-v/4(lcFlag), gapRequest/1, ACC/3(lcFlag)
  Switch/1 -> Scope/2, Min/2  "acc-v"
  ACC-v/1(u) -> Switch/1
  ACC-v/2(errors) -> virtualErrors/1
  ACC-v/3(gap) -> virtualGap/1
  Bus Selector/2 -> Bus Creator/2  "<Y>"
  Signal Specification/1 -> Bus Creator/4, Gain/1
  activate ACC-v/1 -> ACC-v/3(activate), Switch/2
  Constant1/1 -> Switch/3

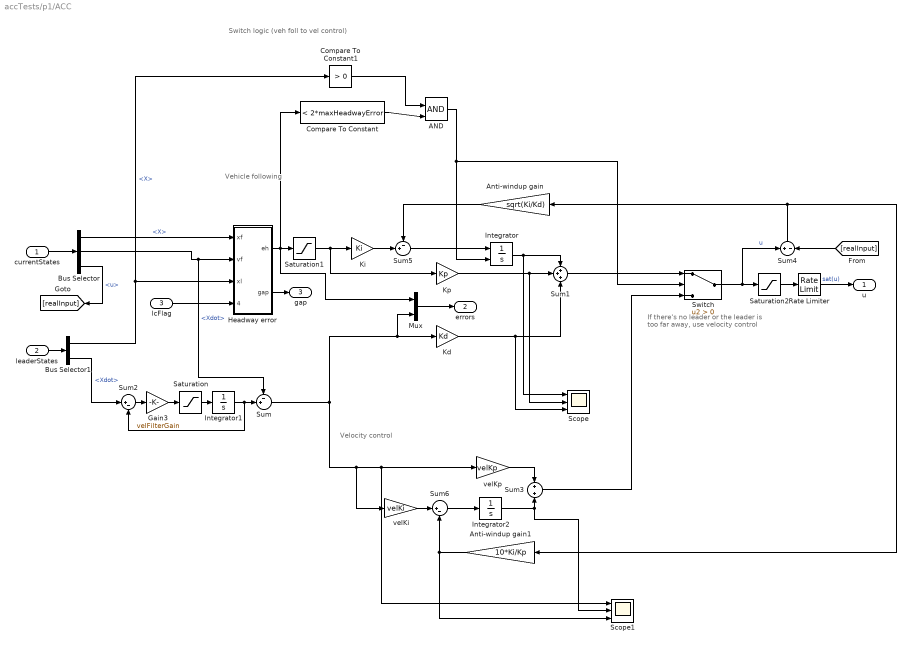
== system accTests/p1/ACC ==
  note: Vehicle following
  note: Switch logic (veh foll to vel control)
  note: Velocity control
  note: If there's no leader or the leader
      | is too far away, use velocity control
  currentStates : Inport
  leaderStates : Inport  Port=2
  lcFlag : Inport  Port=3
  AND : Logic  IconShape=distinctive  AllPortsSameDT=off  OutDataTypeStr=boolean
  Anti-windup gain : Gain  Gain=sqrt(Ki/Kd)
  Anti-windup gain1 : Gain  Gain=10*Ki/Kp
  Bus Selector : BusSelector  OutputSignals=X,Xdot,u
  Bus Selector1 : BusSelector  OutputSignals=X,Xdot
  Compare To Constant : simulink/Logic and Bit Operations/Compare To Constant  relop=<  const=2*maxHeadwayError  OutDataTypeStr=boolean
  Compare To Constant1 : simulink/Logic and Bit Operations/Compare To Constant  relop=>  const=0  OutDataTypeStr=boolean
  Gain3 : Gain  Gain=velFilterGain
  Headway error : Subsystem
  Integrator : Integrator  ExternalReset=either
  Integrator1 : Integrator  InitialCondition=vx0
  Integrator2 : Integrator
  Kd : Gain  Gain=Kd
  Ki : Gain  Gain=Ki
  Kp : Gain  Gain=Kp
  Mux : Mux  Inputs=2
  Rate Limiter : RateLimiter  RisingSlewLimit=maxJerk  FallingSlewLimit=minJerk  SampleTimeMode=inherited
  Saturation : Saturate  UpperLimit=maxAcceleration  LowerLimit=minAcceleration
  Saturation1 : Saturate  UpperLimit=maxHeadwayError  LowerLimit=minHeadwayError
  Saturation2 : Saturate  UpperLimit=maxAcceleration  LowerLimit=minAcceleration
  Scope : Scope  NumInputPorts=3
  Scope1 : Scope  NumInputPorts=3
  Sum : Sum  Inputs=-+|
  Sum1 : Sum  Inputs=+++
  Sum2 : Sum  Inputs=|+-
  Sum3 : Sum
  Sum4 : Sum  Inputs=+-
  Sum5 : Sum  Inputs=-+|
  Sum6 : Sum  Inputs=|+-
  Switch : Switch  Criteria=u2 > Threshold
  velKi : Gain  Gain=velKi
  velKp : Gain  Gain=velKp
  u : Outport
  errors : Outport  Port=2
  gap : Outport  Port=3
  wires:
  Headway error/1(eh) -> Mux/1, Compare To Constant/1, Saturation1/1
  Bus Selector/2 -> Headway error/2(vf), Sum/1  "<Xdot>"
  Kd/1 -> Scope/3, Sum1/3
  Kp/1 -> Scope/2, Sum1/2
  Gain3/1 -> Saturation/1
  Saturation/1 -> Integrator1/1
  Integrator1/1 -> Sum2/2, Sum/2
  Bus Selector1/2 -> Sum2/1  "<Xdot>"
  Sum2/1 -> Gain3/1
  Saturation1/1 -> Kp/1, Ki/1
  Headway error/2("gap ") -> gap/1
  Switch/1 -> Sum4/1, Saturation2/1  "u"
  Sum1/1 -> Switch/1
  Sum3/1 -> Switch/3
  Sum/1 -> Mux/2, Kd/1, velKi/1, Scope1/1, velKp/1
  Mux/1 -> errors/1
  Saturation2/1 -> Rate Limiter/1
  Sum4/1 -> Anti-windup gain/1, Anti-windup gain1/1
  Sum5/1 -> Integrator/1
  Rate Limiter/1 -> u/1  "sat(u)"
  velKp/1 -> Sum3/1
  Ki/1 -> Sum5/2
  Integrator/1 -> Sum1/1, Scope/1
  Anti-windup gain/1 -> Sum5/1
  AND/1 -> Integrator/2, Switch/2
  Compare To Constant/1 -> AND/2
  Compare To Constant1/1 -> AND/1
  lcFlag/1 -> Headway error/4(lcFlag)
  currentStates/1 -> Bus Selector/1
  Bus Selector/1 -> Headway error/1(xf)  "<X>"
  leaderStates/1 -> Bus Selector1/1
  Bus Selector1/1 -> Compare To Constant1/1, Headway error/3(xl)  "<X>"
  Bus Selector/3 -> [realInput]  "<u>"
  [realInput] -> Sum4/2
  Integrator2/1 -> Scope1/2, Sum3/2
  velKi/1 -> Sum6/1
  Sum6/1 -> Integrator2/1
  Anti-windup gain1/1 -> Scope1/3, Sum6/2

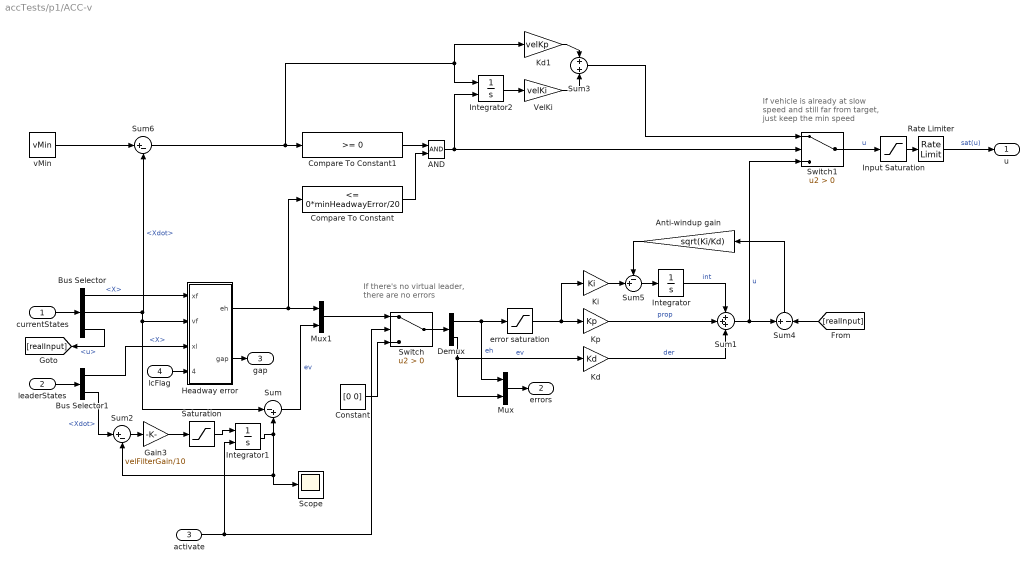
== system accTests/p1/ACC-v ==
  note: If vehicle is already at slow
      | speed and still far from target,
      | just keep the min speed
  note: If there's no virtual leader,
      | there are no errors
  currentStates : Inport
  leaderStates : Inport  Port=2
  activate : Inport  Port=3
  lcFlag : Inport  Port=4
  AND : Logic  IconShape=distinctive  AllPortsSameDT=off  OutDataTypeStr=boolean
  Anti-windup gain : Gain  Gain=sqrt(Ki/Kd)
  Bus Selector : BusSelector  OutputSignals=X,Xdot,u
  Bus Selector1 : BusSelector  OutputSignals=X,Xdot
  Compare To Constant : simulink/Logic and Bit Operations/Compare To Constant  relop=<=  const=0*minHeadwayError/20  OutDataTypeStr=boolean
  Compare To Constant1 : simulink/Logic and Bit Operations/Compare To Constant  relop=>=  const=0  OutDataTypeStr=boolean
  Constant : Constant  Value=[0 0]
  Demux : Demux  Outputs=2
  Gain3 : Gain  Gain=velFilterGain/10
  Headway error : Subsystem
  Input Saturation : Saturate  UpperLimit=maxAcceleration/2  LowerLimit=minAcceleration/4
  Integrator : Integrator
  Integrator1 : Integrator  ExternalReset=rising  InitialCondition=vx0
  Integrator2 : Integrator  ExternalReset=rising
  Kd : Gain  Gain=Kd
  Kd1 : Gain  Gain=velKp
  Ki : Gain  Gain=Ki
  Kp : Gain  Gain=Kp
  Mux : Mux  Inputs=2
  Mux1 : Mux  Inputs=2
  Rate Limiter : RateLimiter  RisingSlewLimit=maxJerk/2  FallingSlewLimit=minJerk/3  SampleTimeMode=inherited
  Saturation : Saturate  UpperLimit=maxAcceleration  LowerLimit=minAcceleration
  Scope : Scope
  Sum : Sum  Inputs=|-+
  Sum1 : Sum  Inputs=+++
  Sum2 : Sum  Inputs=|+-
  Sum3 : Sum
  Sum4 : Sum  Inputs=+-
  Sum5 : Sum  Inputs=-+|
  Sum6 : Sum  Inputs=|+-
  Switch : Switch  Criteria=u2 > Threshold
  Switch1 : Switch  Criteria=u2 > Threshold
  VelKi : Gain  Gain=velKi
  error saturation : Saturate  UpperLimit=maxHeadwayError  LowerLimit=minHeadwayError/10
  vMin : Constant  Value=vMin
  u : Outport
  errors : Outport  Port=2
  gap : Outport  Port=3
  wires:
  Headway error/1(eh) -> Compare To Constant/1, Mux1/1
  Kd/1 -> Sum1/3  "der"
  Kp/1 -> Sum1/2  "prop"
  Gain3/1 -> Saturation/1
  Saturation/1 -> Integrator1/1
  Integrator1/1 -> Scope/1, Sum2/2, Sum/2
  Bus Selector1/2 -> Sum2/1  "<Xdot>"
  Sum2/1 -> Gain3/1
  Demux/1 -> Mux/1, error saturation/1  "eh"
  Headway error/2("gap ") -> gap/1
  Sum1/1 -> Switch1/3, Sum4/1  "u"
  Sum/1 -> Mux1/2  "ev"
  Mux/1 -> errors/1
  Input Saturation/1 -> Rate Limiter/1
  Integrator/1 -> Sum1/1  "int"
  Sum4/1 -> Anti-windup gain/1
  Ki/1 -> Sum5/2
  Anti-windup gain/1 -> Sum5/1
  Demux/2 -> Kd/1, Mux/2  "ev"
  Switch/1 -> Demux/1
  Mux1/1 -> Switch/1
  activate/1 -> Integrator1/2, Switch/2
  Constant/1 -> Switch/3
  Rate Limiter/1 -> u/1  "sat(u)"
  Compare To Constant1/1 -> AND/1
  Compare To Constant/1 -> AND/2
  Sum6/1 -> Integrator2/1, Kd1/1, Compare To Constant1/1
  Sum3/1 -> Switch1/1
  Integrator2/1 -> VelKi/1
  Kd1/1 -> Sum3/1
  VelKi/1 -> Sum3/2
  vMin/1 -> Sum6/1
  Switch1/1 -> Input Saturation/1  "u"
  error saturation/1 -> Kp/1, Ki/1
  Sum5/1 -> Integrator/1
  AND/1 -> Switch1/2, Integrator2/2
  [realInput] -> Sum4/2
  currentStates/1 -> Bus Selector/1
  Bus Selector/1 -> Headway error/1(xf)  "<X>"
  Bus Selector/2 -> Sum6/2, Headway error/2(vf), Sum/1  "<Xdot>"
  leaderStates/1 -> Bus Selector1/1
  Bus Selector1/1 -> Headway error/3(xl)  "<X>"
  Bus Selector/3 -> [realInput]  "<u>"
  lcFlag/1 -> Headway error/4(lcFlag)

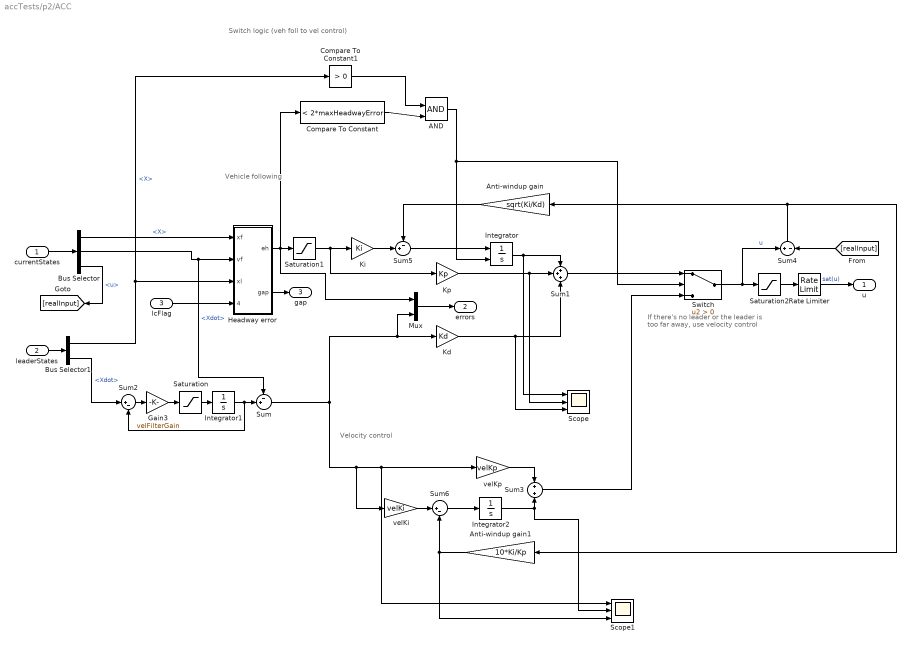
== system accTests/p2/ACC ==
  note: Vehicle following
  note: Switch logic (veh foll to vel control)
  note: Velocity control
  note: If there's no leader or the leader
      | is too far away, use velocity control
  currentStates : Inport
  leaderStates : Inport  Port=2
  lcFlag : Inport  Port=3
  AND : Logic  IconShape=distinctive  AllPortsSameDT=off  OutDataTypeStr=boolean
  Anti-windup gain : Gain  Gain=sqrt(Ki/Kd)
  Anti-windup gain1 : Gain  Gain=10*Ki/Kp
  Bus Selector : BusSelector  OutputSignals=X,Xdot,u
  Bus Selector1 : BusSelector  OutputSignals=X,Xdot
  Compare To Constant : simulink/Logic and Bit Operations/Compare To Constant  relop=<  const=2*maxHeadwayError  OutDataTypeStr=boolean
  Compare To Constant1 : simulink/Logic and Bit Operations/Compare To Constant  relop=>  const=0  OutDataTypeStr=boolean
  Gain3 : Gain  Gain=velFilterGain
  Headway error : Subsystem
  Integrator : Integrator  ExternalReset=either
  Integrator1 : Integrator  InitialCondition=vx0
  Integrator2 : Integrator
  Kd : Gain  Gain=Kd
  Ki : Gain  Gain=Ki
  Kp : Gain  Gain=Kp
  Mux : Mux  Inputs=2
  Rate Limiter : RateLimiter  RisingSlewLimit=maxJerk  FallingSlewLimit=minJerk  SampleTimeMode=inherited
  Saturation : Saturate  UpperLimit=maxAcceleration  LowerLimit=minAcceleration
  Saturation1 : Saturate  UpperLimit=maxHeadwayError  LowerLimit=minHeadwayError
  Saturation2 : Saturate  UpperLimit=maxAcceleration  LowerLimit=minAcceleration
  Scope : Scope  NumInputPorts=3
  Scope1 : Scope  NumInputPorts=3
  Sum : Sum  Inputs=-+|
  Sum1 : Sum  Inputs=+++
  Sum2 : Sum  Inputs=|+-
  Sum3 : Sum
  Sum4 : Sum  Inputs=+-
  Sum5 : Sum  Inputs=-+|
  Sum6 : Sum  Inputs=|+-
  Switch : Switch  Criteria=u2 > Threshold
  velKi : Gain  Gain=velKi
  velKp : Gain  Gain=velKp
  u : Outport
  errors : Outport  Port=2
  gap : Outport  Port=3
  wires:
  Headway error/1(eh) -> Mux/1, Compare To Constant/1, Saturation1/1
  Bus Selector/2 -> Headway error/2(vf), Sum/1  "<Xdot>"
  Kd/1 -> Scope/3, Sum1/3
  Kp/1 -> Scope/2, Sum1/2
  Gain3/1 -> Saturation/1
  Saturation/1 -> Integrator1/1
  Integrator1/1 -> Sum2/2, Sum/2
  Bus Selector1/2 -> Sum2/1  "<Xdot>"
  Sum2/1 -> Gain3/1
  Saturation1/1 -> Kp/1, Ki/1
  Headway error/2("gap ") -> gap/1
  Switch/1 -> Sum4/1, Saturation2/1  "u"
  Sum1/1 -> Switch/1
  Sum3/1 -> Switch/3
  Sum/1 -> Mux/2, Kd/1, velKi/1, Scope1/1, velKp/1
  Mux/1 -> errors/1
  Saturation2/1 -> Rate Limiter/1
  Sum4/1 -> Anti-windup gain/1, Anti-windup gain1/1
  Sum5/1 -> Integrator/1
  Rate Limiter/1 -> u/1  "sat(u)"
  velKp/1 -> Sum3/1
  Ki/1 -> Sum5/2
  Integrator/1 -> Sum1/1, Scope/1
  Anti-windup gain/1 -> Sum5/1
  AND/1 -> Integrator/2, Switch/2
  Compare To Constant/1 -> AND/2
  Compare To Constant1/1 -> AND/1
  lcFlag/1 -> Headway error/4(lcFlag)
  currentStates/1 -> Bus Selector/1
  Bus Selector/1 -> Headway error/1(xf)  "<X>"
  leaderStates/1 -> Bus Selector1/1
  Bus Selector1/1 -> Compare To Constant1/1, Headway error/3(xl)  "<X>"
  Bus Selector/3 -> [realInput]  "<u>"
  [realInput] -> Sum4/2
  Integrator2/1 -> Scope1/2, Sum3/2
  velKi/1 -> Sum6/1
  Sum6/1 -> Integrator2/1
  Anti-windup gain1/1 -> Scope1/3, Sum6/2

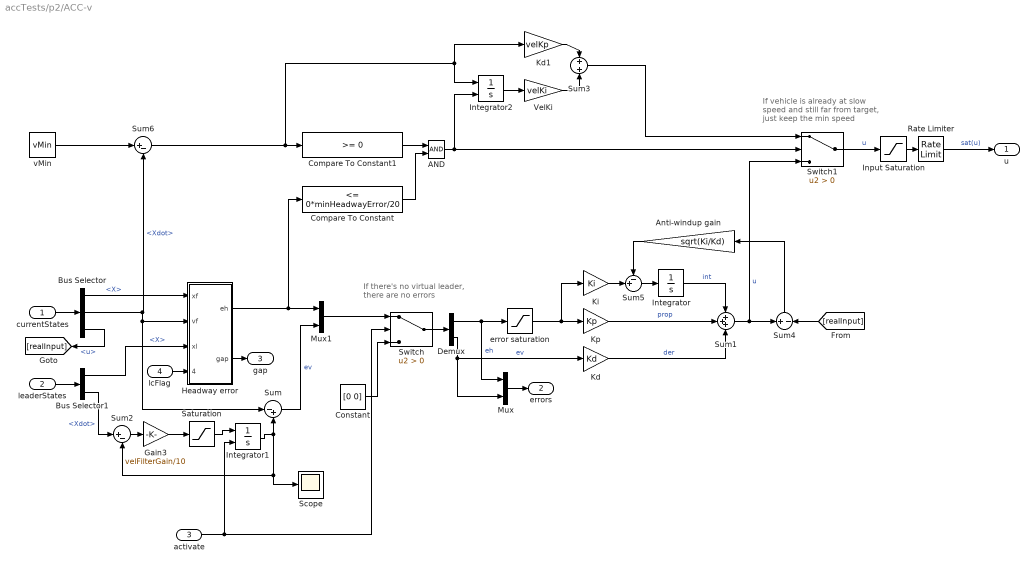
== system accTests/p2/ACC-v ==
  note: If vehicle is already at slow
      | speed and still far from target,
      | just keep the min speed
  note: If there's no virtual leader,
      | there are no errors
  currentStates : Inport
  leaderStates : Inport  Port=2
  activate : Inport  Port=3
  lcFlag : Inport  Port=4
  AND : Logic  IconShape=distinctive  AllPortsSameDT=off  OutDataTypeStr=boolean
  Anti-windup gain : Gain  Gain=sqrt(Ki/Kd)
  Bus Selector : BusSelector  OutputSignals=X,Xdot,u
  Bus Selector1 : BusSelector  OutputSignals=X,Xdot
  Compare To Constant : simulink/Logic and Bit Operations/Compare To Constant  relop=<=  const=0*minHeadwayError/20  OutDataTypeStr=boolean
  Compare To Constant1 : simulink/Logic and Bit Operations/Compare To Constant  relop=>=  const=0  OutDataTypeStr=boolean
  Constant : Constant  Value=[0 0]
  Demux : Demux  Outputs=2
  Gain3 : Gain  Gain=velFilterGain/10
  Headway error : Subsystem
  Input Saturation : Saturate  UpperLimit=maxAcceleration/2  LowerLimit=minAcceleration/4
  Integrator : Integrator
  Integrator1 : Integrator  ExternalReset=rising  InitialCondition=vx0
  Integrator2 : Integrator  ExternalReset=rising
  Kd : Gain  Gain=Kd
  Kd1 : Gain  Gain=velKp
  Ki : Gain  Gain=Ki
  Kp : Gain  Gain=Kp
  Mux : Mux  Inputs=2
  Mux1 : Mux  Inputs=2
  Rate Limiter : RateLimiter  RisingSlewLimit=maxJerk/2  FallingSlewLimit=minJerk/3  SampleTimeMode=inherited
  Saturation : Saturate  UpperLimit=maxAcceleration  LowerLimit=minAcceleration
  Scope : Scope
  Sum : Sum  Inputs=|-+
  Sum1 : Sum  Inputs=+++
  Sum2 : Sum  Inputs=|+-
  Sum3 : Sum
  Sum4 : Sum  Inputs=+-
  Sum5 : Sum  Inputs=-+|
  Sum6 : Sum  Inputs=|+-
  Switch : Switch  Criteria=u2 > Threshold
  Switch1 : Switch  Criteria=u2 > Threshold
  VelKi : Gain  Gain=velKi
  error saturation : Saturate  UpperLimit=maxHeadwayError  LowerLimit=minHeadwayError/10
  vMin : Constant  Value=vMin
  u : Outport
  errors : Outport  Port=2
  gap : Outport  Port=3
  wires:
  Headway error/1(eh) -> Compare To Constant/1, Mux1/1
  Kd/1 -> Sum1/3  "der"
  Kp/1 -> Sum1/2  "prop"
  Gain3/1 -> Saturation/1
  Saturation/1 -> Integrator1/1
  Integrator1/1 -> Scope/1, Sum2/2, Sum/2
  Bus Selector1/2 -> Sum2/1  "<Xdot>"
  Sum2/1 -> Gain3/1
  Demux/1 -> Mux/1, error saturation/1  "eh"
  Headway error/2("gap ") -> gap/1
  Sum1/1 -> Switch1/3, Sum4/1  "u"
  Sum/1 -> Mux1/2  "ev"
  Mux/1 -> errors/1
  Input Saturation/1 -> Rate Limiter/1
  Integrator/1 -> Sum1/1  "int"
  Sum4/1 -> Anti-windup gain/1
  Ki/1 -> Sum5/2
  Anti-windup gain/1 -> Sum5/1
  Demux/2 -> Kd/1, Mux/2  "ev"
  Switch/1 -> Demux/1
  Mux1/1 -> Switch/1
  activate/1 -> Integrator1/2, Switch/2
  Constant/1 -> Switch/3
  Rate Limiter/1 -> u/1  "sat(u)"
  Compare To Constant1/1 -> AND/1
  Compare To Constant/1 -> AND/2
  Sum6/1 -> Integrator2/1, Kd1/1, Compare To Constant1/1
  Sum3/1 -> Switch1/1
  Integrator2/1 -> VelKi/1
  Kd1/1 -> Sum3/1
  VelKi/1 -> Sum3/2
  vMin/1 -> Sum6/1
  Switch1/1 -> Input Saturation/1  "u"
  error saturation/1 -> Kp/1, Ki/1
  Sum5/1 -> Integrator/1
  AND/1 -> Switch1/2, Integrator2/2
  [realInput] -> Sum4/2
  currentStates/1 -> Bus Selector/1
  Bus Selector/1 -> Headway error/1(xf)  "<X>"
  Bus Selector/2 -> Sum6/2, Headway error/2(vf), Sum/1  "<Xdot>"
  leaderStates/1 -> Bus Selector1/1
  Bus Selector1/1 -> Headway error/3(xl)  "<X>"
  Bus Selector/3 -> [realInput]  "<u>"
  lcFlag/1 -> Headway error/4(lcFlag)

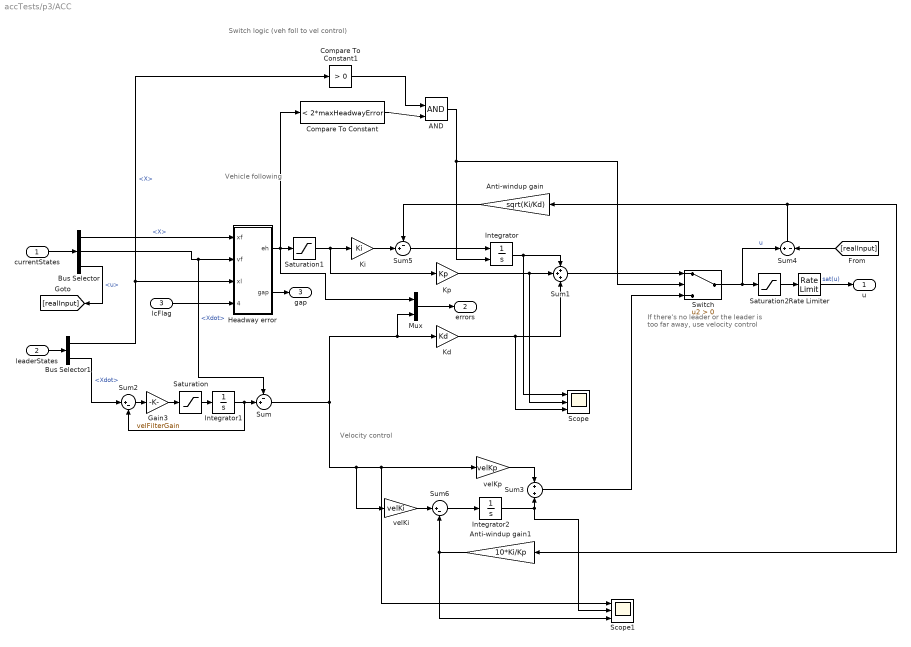
== system accTests/p3/ACC ==
  note: Vehicle following
  note: Switch logic (veh foll to vel control)
  note: Velocity control
  note: If there's no leader or the leader
      | is too far away, use velocity control
  currentStates : Inport
  leaderStates : Inport  Port=2
  lcFlag : Inport  Port=3
  AND : Logic  IconShape=distinctive  AllPortsSameDT=off  OutDataTypeStr=boolean
  Anti-windup gain : Gain  Gain=sqrt(Ki/Kd)
  Anti-windup gain1 : Gain  Gain=10*Ki/Kp
  Bus Selector : BusSelector  OutputSignals=X,Xdot,u
  Bus Selector1 : BusSelector  OutputSignals=X,Xdot
  Compare To Constant : simulink/Logic and Bit Operations/Compare To Constant  relop=<  const=2*maxHeadwayError  OutDataTypeStr=boolean
  Compare To Constant1 : simulink/Logic and Bit Operations/Compare To Constant  relop=>  const=0  OutDataTypeStr=boolean
  Gain3 : Gain  Gain=velFilterGain
  Headway error : Subsystem
  Integrator : Integrator  ExternalReset=either
  Integrator1 : Integrator  InitialCondition=vx0
  Integrator2 : Integrator
  Kd : Gain  Gain=Kd
  Ki : Gain  Gain=Ki
  Kp : Gain  Gain=Kp
  Mux : Mux  Inputs=2
  Rate Limiter : RateLimiter  RisingSlewLimit=maxJerk  FallingSlewLimit=minJerk  SampleTimeMode=inherited
  Saturation : Saturate  UpperLimit=maxAcceleration  LowerLimit=minAcceleration
  Saturation1 : Saturate  UpperLimit=maxHeadwayError  LowerLimit=minHeadwayError
  Saturation2 : Saturate  UpperLimit=maxAcceleration  LowerLimit=minAcceleration
  Scope : Scope  NumInputPorts=3
  Scope1 : Scope  NumInputPorts=3
  Sum : Sum  Inputs=-+|
  Sum1 : Sum  Inputs=+++
  Sum2 : Sum  Inputs=|+-
  Sum3 : Sum
  Sum4 : Sum  Inputs=+-
  Sum5 : Sum  Inputs=-+|
  Sum6 : Sum  Inputs=|+-
  Switch : Switch  Criteria=u2 > Threshold
  velKi : Gain  Gain=velKi
  velKp : Gain  Gain=velKp
  u : Outport
  errors : Outport  Port=2
  gap : Outport  Port=3
  wires:
  Headway error/1(eh) -> Mux/1, Compare To Constant/1, Saturation1/1
  Bus Selector/2 -> Headway error/2(vf), Sum/1  "<Xdot>"
  Kd/1 -> Scope/3, Sum1/3
  Kp/1 -> Scope/2, Sum1/2
  Gain3/1 -> Saturation/1
  Saturation/1 -> Integrator1/1
  Integrator1/1 -> Sum2/2, Sum/2
  Bus Selector1/2 -> Sum2/1  "<Xdot>"
  Sum2/1 -> Gain3/1
  Saturation1/1 -> Kp/1, Ki/1
  Headway error/2("gap ") -> gap/1
  Switch/1 -> Sum4/1, Saturation2/1  "u"
  Sum1/1 -> Switch/1
  Sum3/1 -> Switch/3
  Sum/1 -> Mux/2, Kd/1, velKi/1, Scope1/1, velKp/1
  Mux/1 -> errors/1
  Saturation2/1 -> Rate Limiter/1
  Sum4/1 -> Anti-windup gain/1, Anti-windup gain1/1
  Sum5/1 -> Integrator/1
  Rate Limiter/1 -> u/1  "sat(u)"
  velKp/1 -> Sum3/1
  Ki/1 -> Sum5/2
  Integrator/1 -> Sum1/1, Scope/1
  Anti-windup gain/1 -> Sum5/1
  AND/1 -> Integrator/2, Switch/2
  Compare To Constant/1 -> AND/2
  Compare To Constant1/1 -> AND/1
  lcFlag/1 -> Headway error/4(lcFlag)
  currentStates/1 -> Bus Selector/1
  Bus Selector/1 -> Headway error/1(xf)  "<X>"
  leaderStates/1 -> Bus Selector1/1
  Bus Selector1/1 -> Compare To Constant1/1, Headway error/3(xl)  "<X>"
  Bus Selector/3 -> [realInput]  "<u>"
  [realInput] -> Sum4/2
  Integrator2/1 -> Scope1/2, Sum3/2
  velKi/1 -> Sum6/1
  Sum6/1 -> Integrator2/1
  Anti-windup gain1/1 -> Scope1/3, Sum6/2
